simulink model "dpsk"  (R2018b)
settings: Solver=VariableStepAuto  StartTime=0.0  StopTime=10.0  RelTol=1e-3
libraries: dsparch4 x2, commrandsrc3 x1, commsrccod2 x1, commutil2 x1
settings Model: Creator=86138  LastModifiedBy=86138

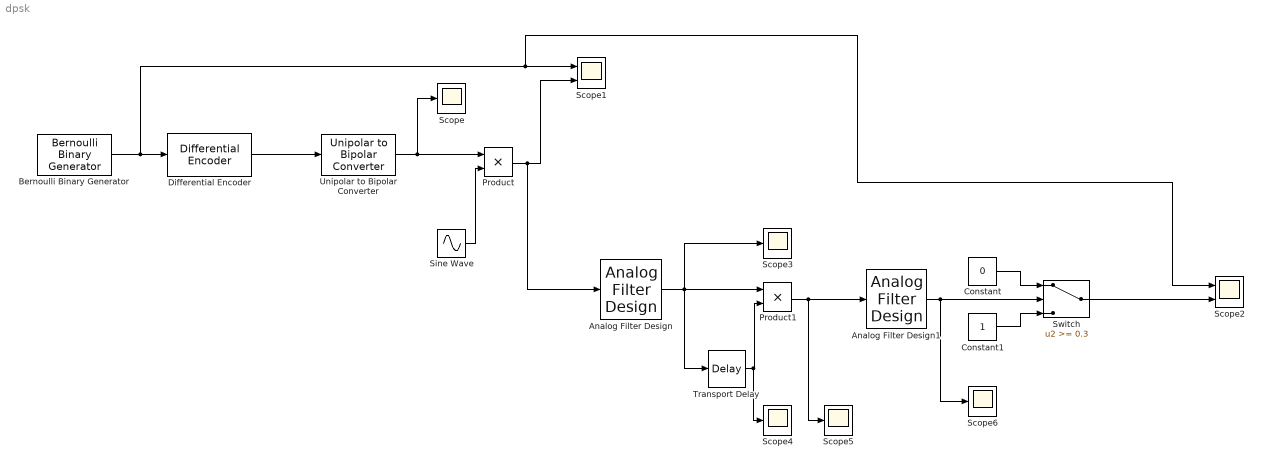
== system dpsk ==
  Analog Filter Design : dsparch4/Analog Filter Design  method=Butterworth  filttype=Bandpass  N=8  Wlo=2*2*pi  Whi=7*2*pi  Rp=2  Rs=40
  Analog Filter Design1 : dsparch4/Analog Filter Design  method=Butterworth  filttype=Lowpass  N=4  Wlo=3*2*pi  Whi=80  Rp=2  Rs=40
  Bernoulli Binary Generator : commrandsrc3/Bernoulli Binary Generator  ProbabilityOfZero=0.5  SeedSource=Auto  Seed=0  SampleTime=1  SamplesPerFrame=1  OutputDataType=double  SimulateUsing=Interpreted execution
  Constant : Constant  Value=0
  Constant1 : Constant
  Differential Encoder : commsrccod2/Differential Encoder  InitCond=0.05
      settings: SourceProductName=Communications System Toolbox  SourceProductBaseCode=CM
  Product : Product
  Product1 : Product
  Scope{,3..6} (5 alike) : Scope
  Scope1 : Scope  NumInputPorts=2
  Scope2 : Scope  NumInputPorts=2
  Sine Wave : Sin  Amplitude=2  Frequency=4*2*pi  SampleTime=1/500
  Switch : Switch  Threshold=0.3
  Transport Delay : TransportDelay  DelayTime=0.318*pi
  Unipolar to Bipolar Converter : commutil2/Unipolar to Bipolar Converter  M=2  polarity=Positive  dataType=Same as input
      settings: SourceProductName=Communications System Toolbox
  wires:
  Bernoulli Binary Generator/1 -> Scope2/1, Scope1/1, Differential Encoder/1
  Differential Encoder/1 -> Unipolar to Bipolar Converter/1
  Unipolar to Bipolar Converter/1 -> Product/1, Scope/1
  Sine Wave/1 -> Product/2
  Product/1 -> Analog Filter Design/1, Scope1/2
  Analog Filter Design/1 -> Scope3/1, Product1/1, Transport Delay/1
  Transport Delay/1 -> Scope4/1, Product1/2
  Product1/1 -> Scope5/1, Analog Filter Design1/1
  Analog Filter Design1/1 -> Scope6/1, Switch/2
  Constant/1 -> Switch/1
  Constant1/1 -> Switch/3
  Switch/1 -> Scope2/2
